simulink model "gm_DSBF"  (R2019b)
settings: Solver=FixedStepDiscrete  StartTime=0.0  StopTime=0.02  RelTol=1e-3
InitFcn:
  | sm_callback_init
StopFcn:
  | sm_callback_stop
undefined symbols (not defined in the file or in its folder): arraySize, arraySpacing, delayDataTypeFractionLength, delayDataTypeSign, delayDataTypeWordLength, mp, samplingRate, speedOfSound, upsampleFactor
libraries: hdlsllib x64, simulink x36, dspmlti4 x16, dsphdlfiltering x16
(part 4 of 5)

== system gm_DSBF/dataplane/Avalon Data Processing/delay signals_instance12/delay signal/read address generator ==
  note: To accommodate positive and negative delays, the read pointer needs to lag the write pointer by the maximum delay + 1. For the maximum positive delay, this puts the read pointer 1 behind the write pointer.
  note: this offset is the maximum possible delay from a microphone to the the center of the array
  note: wrap on overflow is the desired behavior
  write_addr : Inport  OutDataTypeStr=fixdt(0, 6, 0)  PortDimensions=1  SampleTime=2.08333333333333e-05
  delay : Inport  Port=2  OutDataTypeStr=fixdt(1, 6, 0)  PortDimensions=1  SampleTime=2.08333333333333e-05
  Increment Real World : simulink/Additional Math & Discrete/Additional Math: Increment - Decrement/Increment Real World
      settings: SourceProductName=Simulink  SourceProductBaseCode=SL
  Subtract : Subsystem
  phase center reference offset : Constant  Value=fix(mp.maxDelay/2)  OutDataTypeStr=fixdt(0,delayDataTypeWordLength - delayDataTypeFractionLength,0)  SampleTime=-1
  read_addr : Outport  VectorParamsAs1DForOutWhenUnconnected=off
  wires:
  delay/1 -> Subtract/1(In1)
  write_addr/1 -> Subtract/2(In2)
  Increment Real World/1 -> Subtract/3(In3)
  Subtract/1(Out1) -> read_addr/1
  phase center reference offset/1 -> Increment Real World/1

== system gm_DSBF/dataplane/Avalon Data Processing/delay signals_instance12/delay signal/read address generator1 ==
  note: wrap on overflow is the desired behavior
  note: To accommodate positive and negative delays, the read pointer needs to lag the write pointer by the maximum delay + 1. For the maximum positive delay, this puts the read pointer 1 behind the write pointer.
  note: this offset is the maximum possible delay from a microphone to the the center of the array
  write_addr : Inport  OutDataTypeStr=fixdt(0, 6, 0)  PortDimensions=1  SampleTime=1.30208333333333e-06
  delay : Inport  Port=2  OutDataTypeStr=fixdt(1, 6, 0)  PortDimensions=1  SampleTime=1.30208333333333e-06
  Increment Real World : simulink/Additional Math & Discrete/Additional Math: Increment - Decrement/Increment Real World
      settings: SourceProductName=Simulink  SourceProductBaseCode=SL
  Subtract : Subsystem
  phase center reference offset : Constant  Value=fix(mp.upsampleFactor)  OutDataTypeStr=fixdt(0, delayDataTypeFractionLength, 0)  SampleTime=-1
  read_addr : Outport  VectorParamsAs1DForOutWhenUnconnected=off
  wires:
  delay/1 -> Subtract/1(In1)
  write_addr/1 -> Subtract/2(In2)
  Increment Real World/1 -> Subtract/3(In3)
  Subtract/1(Out1) -> read_addr/1
  phase center reference offset/1 -> Increment Real World/1

== system gm_DSBF/dataplane/Avalon Data Processing/delay signals_instance12/delay signal/split_into_int_and_frac_parts ==
  delay : Inport  OutDataTypeStr=fixdt(1, 12, 6)  PortDimensions=1  SampleTime=2.08333333333333e-05
  split_into_int_and_frac_parts : MATLAB Function  TreatAsAtomicUnit=on
  integer_delay : Outport  VectorParamsAs1DForOutWhenUnconnected=off
  fractional_delay : Outport  Port=2
  wires:
  delay/1 -> split_into_int_and_frac_parts/1(delay)
  split_into_int_and_frac_parts/2(fractional_delay) -> fractional_delay/1
  split_into_int_and_frac_parts/1(integer_delay) -> integer_delay/1

== system gm_DSBF/dataplane/Avalon Data Processing/delay signals_instance13/delay signal/read address generator ==
  note: To accommodate positive and negative delays, the read pointer needs to lag the write pointer by the maximum delay + 1. For the maximum positive delay, this puts the read pointer 1 behind the write pointer.
  note: this offset is the maximum possible delay from a microphone to the the center of the array
  note: wrap on overflow is the desired behavior
  write_addr : Inport  OutDataTypeStr=fixdt(0, 6, 0)  PortDimensions=1  SampleTime=2.08333333333333e-05
  delay : Inport  Port=2  OutDataTypeStr=fixdt(1, 6, 0)  PortDimensions=1  SampleTime=2.08333333333333e-05
  Increment Real World : simulink/Additional Math & Discrete/Additional Math: Increment - Decrement/Increment Real World
      settings: SourceProductName=Simulink  SourceProductBaseCode=SL
  Subtract : Subsystem
  phase center reference offset : Constant  Value=fix(mp.maxDelay/2)  OutDataTypeStr=fixdt(0,delayDataTypeWordLength - delayDataTypeFractionLength,0)  SampleTime=-1
  read_addr : Outport  VectorParamsAs1DForOutWhenUnconnected=off
  wires:
  delay/1 -> Subtract/1(In1)
  write_addr/1 -> Subtract/2(In2)
  Increment Real World/1 -> Subtract/3(In3)
  Subtract/1(Out1) -> read_addr/1
  phase center reference offset/1 -> Increment Real World/1

== system gm_DSBF/dataplane/Avalon Data Processing/delay signals_instance13/delay signal/read address generator1 ==
  note: wrap on overflow is the desired behavior
  note: To accommodate positive and negative delays, the read pointer needs to lag the write pointer by the maximum delay + 1. For the maximum positive delay, this puts the read pointer 1 behind the write pointer.
  note: this offset is the maximum possible delay from a microphone to the the center of the array
  write_addr : Inport  OutDataTypeStr=fixdt(0, 6, 0)  PortDimensions=1  SampleTime=1.30208333333333e-06
  delay : Inport  Port=2  OutDataTypeStr=fixdt(1, 6, 0)  PortDimensions=1  SampleTime=1.30208333333333e-06
  Increment Real World : simulink/Additional Math & Discrete/Additional Math: Increment - Decrement/Increment Real World
      settings: SourceProductName=Simulink  SourceProductBaseCode=SL
  Subtract : Subsystem
  phase center reference offset : Constant  Value=fix(mp.upsampleFactor)  OutDataTypeStr=fixdt(0, delayDataTypeFractionLength, 0)  SampleTime=-1
  read_addr : Outport  VectorParamsAs1DForOutWhenUnconnected=off
  wires:
  delay/1 -> Subtract/1(In1)
  write_addr/1 -> Subtract/2(In2)
  Increment Real World/1 -> Subtract/3(In3)
  Subtract/1(Out1) -> read_addr/1
  phase center reference offset/1 -> Increment Real World/1

== system gm_DSBF/dataplane/Avalon Data Processing/delay signals_instance13/delay signal/split_into_int_and_frac_parts ==
  delay : Inport  OutDataTypeStr=fixdt(1, 12, 6)  PortDimensions=1  SampleTime=2.08333333333333e-05
  split_into_int_and_frac_parts : MATLAB Function  TreatAsAtomicUnit=on
  integer_delay : Outport  VectorParamsAs1DForOutWhenUnconnected=off
  fractional_delay : Outport  Port=2
  wires:
  delay/1 -> split_into_int_and_frac_parts/1(delay)
  split_into_int_and_frac_parts/2(fractional_delay) -> fractional_delay/1
  split_into_int_and_frac_parts/1(integer_delay) -> integer_delay/1

== system gm_DSBF/dataplane/Avalon Data Processing/delay signals_instance14/delay signal/read address generator ==
  note: To accommodate positive and negative delays, the read pointer needs to lag the write pointer by the maximum delay + 1. For the maximum positive delay, this puts the read pointer 1 behind the write pointer.
  note: this offset is the maximum possible delay from a microphone to the the center of the array
  note: wrap on overflow is the desired behavior
  write_addr : Inport  OutDataTypeStr=fixdt(0, 6, 0)  PortDimensions=1  SampleTime=2.08333333333333e-05
  delay : Inport  Port=2  OutDataTypeStr=fixdt(1, 6, 0)  PortDimensions=1  SampleTime=2.08333333333333e-05
  Increment Real World : simulink/Additional Math & Discrete/Additional Math: Increment - Decrement/Increment Real World
      settings: SourceProductName=Simulink  SourceProductBaseCode=SL
  Subtract : Subsystem
  phase center reference offset : Constant  Value=fix(mp.maxDelay/2)  OutDataTypeStr=fixdt(0,delayDataTypeWordLength - delayDataTypeFractionLength,0)  SampleTime=-1
  read_addr : Outport  VectorParamsAs1DForOutWhenUnconnected=off
  wires:
  delay/1 -> Subtract/1(In1)
  write_addr/1 -> Subtract/2(In2)
  Increment Real World/1 -> Subtract/3(In3)
  Subtract/1(Out1) -> read_addr/1
  phase center reference offset/1 -> Increment Real World/1

== system gm_DSBF/dataplane/Avalon Data Processing/delay signals_instance14/delay signal/read address generator1 ==
  note: wrap on overflow is the desired behavior
  note: To accommodate positive and negative delays, the read pointer needs to lag the write pointer by the maximum delay + 1. For the maximum positive delay, this puts the read pointer 1 behind the write pointer.
  note: this offset is the maximum possible delay from a microphone to the the center of the array
  write_addr : Inport  OutDataTypeStr=fixdt(0, 6, 0)  PortDimensions=1  SampleTime=1.30208333333333e-06
  delay : Inport  Port=2  OutDataTypeStr=fixdt(1, 6, 0)  PortDimensions=1  SampleTime=1.30208333333333e-06
  Increment Real World : simulink/Additional Math & Discrete/Additional Math: Increment - Decrement/Increment Real World
      settings: SourceProductName=Simulink  SourceProductBaseCode=SL
  Subtract : Subsystem
  phase center reference offset : Constant  Value=fix(mp.upsampleFactor)  OutDataTypeStr=fixdt(0, delayDataTypeFractionLength, 0)  SampleTime=-1
  read_addr : Outport  VectorParamsAs1DForOutWhenUnconnected=off
  wires:
  delay/1 -> Subtract/1(In1)
  write_addr/1 -> Subtract/2(In2)
  Increment Real World/1 -> Subtract/3(In3)
  Subtract/1(Out1) -> read_addr/1
  phase center reference offset/1 -> Increment Real World/1

== system gm_DSBF/dataplane/Avalon Data Processing/delay signals_instance14/delay signal/split_into_int_and_frac_parts ==
  delay : Inport  OutDataTypeStr=fixdt(1, 12, 6)  PortDimensions=1  SampleTime=2.08333333333333e-05
  split_into_int_and_frac_parts : MATLAB Function  TreatAsAtomicUnit=on
  integer_delay : Outport  VectorParamsAs1DForOutWhenUnconnected=off
  fractional_delay : Outport  Port=2
  wires:
  delay/1 -> split_into_int_and_frac_parts/1(delay)
  split_into_int_and_frac_parts/2(fractional_delay) -> fractional_delay/1
  split_into_int_and_frac_parts/1(integer_delay) -> integer_delay/1

== system gm_DSBF/dataplane/Avalon Data Processing/delay signals_instance15/delay signal/read address generator ==
  note: To accommodate positive and negative delays, the read pointer needs to lag the write pointer by the maximum delay + 1. For the maximum positive delay, this puts the read pointer 1 behind the write pointer.
  note: this offset is the maximum possible delay from a microphone to the the center of the array
  note: wrap on overflow is the desired behavior
  write_addr : Inport  OutDataTypeStr=fixdt(0, 6, 0)  PortDimensions=1  SampleTime=2.08333333333333e-05
  delay : Inport  Port=2  OutDataTypeStr=fixdt(1, 6, 0)  PortDimensions=1  SampleTime=2.08333333333333e-05
  Increment Real World : simulink/Additional Math & Discrete/Additional Math: Increment - Decrement/Increment Real World
      settings: SourceProductName=Simulink  SourceProductBaseCode=SL
  Subtract : Subsystem
  phase center reference offset : Constant  Value=fix(mp.maxDelay/2)  OutDataTypeStr=fixdt(0,delayDataTypeWordLength - delayDataTypeFractionLength,0)  SampleTime=-1
  read_addr : Outport  VectorParamsAs1DForOutWhenUnconnected=off
  wires:
  delay/1 -> Subtract/1(In1)
  write_addr/1 -> Subtract/2(In2)
  Increment Real World/1 -> Subtract/3(In3)
  Subtract/1(Out1) -> read_addr/1
  phase center reference offset/1 -> Increment Real World/1

== system gm_DSBF/dataplane/Avalon Data Processing/delay signals_instance15/delay signal/read address generator1 ==
  note: wrap on overflow is the desired behavior
  note: To accommodate positive and negative delays, the read pointer needs to lag the write pointer by the maximum delay + 1. For the maximum positive delay, this puts the read pointer 1 behind the write pointer.
  note: this offset is the maximum possible delay from a microphone to the the center of the array
  write_addr : Inport  OutDataTypeStr=fixdt(0, 6, 0)  PortDimensions=1  SampleTime=1.30208333333333e-06
  delay : Inport  Port=2  OutDataTypeStr=fixdt(1, 6, 0)  PortDimensions=1  SampleTime=1.30208333333333e-06
  Increment Real World : simulink/Additional Math & Discrete/Additional Math: Increment - Decrement/Increment Real World
      settings: SourceProductName=Simulink  SourceProductBaseCode=SL
  Subtract : Subsystem
  phase center reference offset : Constant  Value=fix(mp.upsampleFactor)  OutDataTypeStr=fixdt(0, delayDataTypeFractionLength, 0)  SampleTime=-1
  read_addr : Outport  VectorParamsAs1DForOutWhenUnconnected=off
  wires:
  delay/1 -> Subtract/1(In1)
  write_addr/1 -> Subtract/2(In2)
  Increment Real World/1 -> Subtract/3(In3)
  Subtract/1(Out1) -> read_addr/1
  phase center reference offset/1 -> Increment Real World/1

== system gm_DSBF/dataplane/Avalon Data Processing/delay signals_instance15/delay signal/split_into_int_and_frac_parts ==
  delay : Inport  OutDataTypeStr=fixdt(1, 12, 6)  PortDimensions=1  SampleTime=2.08333333333333e-05
  split_into_int_and_frac_parts : MATLAB Function  TreatAsAtomicUnit=on
  integer_delay : Outport  VectorParamsAs1DForOutWhenUnconnected=off
  fractional_delay : Outport  Port=2
  wires:
  delay/1 -> split_into_int_and_frac_parts/1(delay)
  split_into_int_and_frac_parts/2(fractional_delay) -> fractional_delay/1
  split_into_int_and_frac_parts/1(integer_delay) -> integer_delay/1

== system gm_DSBF/dataplane/Avalon Data Processing/delay signals_instance16/delay signal/read address generator ==
  note: To accommodate positive and negative delays, the read pointer needs to lag the write pointer by the maximum delay + 1. For the maximum positive delay, this puts the read pointer 1 behind the write pointer.
  note: this offset is the maximum possible delay from a microphone to the the center of the array
  note: wrap on overflow is the desired behavior
  write_addr : Inport  OutDataTypeStr=fixdt(0, 6, 0)  PortDimensions=1  SampleTime=2.08333333333333e-05
  delay : Inport  Port=2  OutDataTypeStr=fixdt(1, 6, 0)  PortDimensions=1  SampleTime=2.08333333333333e-05
  Increment Real World : simulink/Additional Math & Discrete/Additional Math: Increment - Decrement/Increment Real World
      settings: SourceProductName=Simulink  SourceProductBaseCode=SL
  Subtract : Subsystem
  phase center reference offset : Constant  Value=fix(mp.maxDelay/2)  OutDataTypeStr=fixdt(0,delayDataTypeWordLength - delayDataTypeFractionLength,0)  SampleTime=-1
  read_addr : Outport  VectorParamsAs1DForOutWhenUnconnected=off
  wires:
  delay/1 -> Subtract/1(In1)
  write_addr/1 -> Subtract/2(In2)
  Increment Real World/1 -> Subtract/3(In3)
  Subtract/1(Out1) -> read_addr/1
  phase center reference offset/1 -> Increment Real World/1

== system gm_DSBF/dataplane/Avalon Data Processing/delay signals_instance16/delay signal/read address generator1 ==
  note: wrap on overflow is the desired behavior
  note: To accommodate positive and negative delays, the read pointer needs to lag the write pointer by the maximum delay + 1. For the maximum positive delay, this puts the read pointer 1 behind the write pointer.
  note: this offset is the maximum possible delay from a microphone to the the center of the array
  write_addr : Inport  OutDataTypeStr=fixdt(0, 6, 0)  PortDimensions=1  SampleTime=1.30208333333333e-06
  delay : Inport  Port=2  OutDataTypeStr=fixdt(1, 6, 0)  PortDimensions=1  SampleTime=1.30208333333333e-06
  Increment Real World : simulink/Additional Math & Discrete/Additional Math: Increment - Decrement/Increment Real World
      settings: SourceProductName=Simulink  SourceProductBaseCode=SL
  Subtract : Subsystem
  phase center reference offset : Constant  Value=fix(mp.upsampleFactor)  OutDataTypeStr=fixdt(0, delayDataTypeFractionLength, 0)  SampleTime=-1
  read_addr : Outport  VectorParamsAs1DForOutWhenUnconnected=off
  wires:
  delay/1 -> Subtract/1(In1)
  write_addr/1 -> Subtract/2(In2)
  Increment Real World/1 -> Subtract/3(In3)
  Subtract/1(Out1) -> read_addr/1
  phase center reference offset/1 -> Increment Real World/1

== system gm_DSBF/dataplane/Avalon Data Processing/delay signals_instance16/delay signal/split_into_int_and_frac_parts ==
  delay : Inport  OutDataTypeStr=fixdt(1, 12, 6)  PortDimensions=1  SampleTime=2.08333333333333e-05
  split_into_int_and_frac_parts : MATLAB Function  TreatAsAtomicUnit=on
  integer_delay : Outport  VectorParamsAs1DForOutWhenUnconnected=off
  fractional_delay : Outport  Port=2
  wires:
  delay/1 -> split_into_int_and_frac_parts/1(delay)
  split_into_int_and_frac_parts/2(fractional_delay) -> fractional_delay/1
  split_into_int_and_frac_parts/1(integer_delay) -> integer_delay/1

== system gm_DSBF/dataplane/Avalon Data Processing/delay signals_instance2/delay signal/read address generator ==
  note: To accommodate positive and negative delays, the read pointer needs to lag the write pointer by the maximum delay + 1. For the maximum positive delay, this puts the read pointer 1 behind the write pointer.
  note: this offset is the maximum possible delay from a microphone to the the center of the array
  note: wrap on overflow is the desired behavior
  write_addr : Inport  OutDataTypeStr=fixdt(0, 6, 0)  PortDimensions=1  SampleTime=2.08333333333333e-05
  delay : Inport  Port=2  OutDataTypeStr=fixdt(1, 6, 0)  PortDimensions=1  SampleTime=2.08333333333333e-05
  Increment Real World : simulink/Additional Math & Discrete/Additional Math: Increment - Decrement/Increment Real World
      settings: SourceProductName=Simulink  SourceProductBaseCode=SL
  Subtract : Subsystem
  phase center reference offset : Constant  Value=fix(mp.maxDelay/2)  OutDataTypeStr=fixdt(0,delayDataTypeWordLength - delayDataTypeFractionLength,0)  SampleTime=-1
  read_addr : Outport  VectorParamsAs1DForOutWhenUnconnected=off
  wires:
  delay/1 -> Subtract/1(In1)
  write_addr/1 -> Subtract/2(In2)
  Increment Real World/1 -> Subtract/3(In3)
  Subtract/1(Out1) -> read_addr/1
  phase center reference offset/1 -> Increment Real World/1

== system gm_DSBF/dataplane/Avalon Data Processing/delay signals_instance2/delay signal/read address generator1 ==
  note: wrap on overflow is the desired behavior
  note: To accommodate positive and negative delays, the read pointer needs to lag the write pointer by the maximum delay + 1. For the maximum positive delay, this puts the read pointer 1 behind the write pointer.
  note: this offset is the maximum possible delay from a microphone to the the center of the array
  write_addr : Inport  OutDataTypeStr=fixdt(0, 6, 0)  PortDimensions=1  SampleTime=1.30208333333333e-06
  delay : Inport  Port=2  OutDataTypeStr=fixdt(1, 6, 0)  PortDimensions=1  SampleTime=1.30208333333333e-06
  Increment Real World : simulink/Additional Math & Discrete/Additional Math: Increment - Decrement/Increment Real World
      settings: SourceProductName=Simulink  SourceProductBaseCode=SL
  Subtract : Subsystem
  phase center reference offset : Constant  Value=fix(mp.upsampleFactor)  OutDataTypeStr=fixdt(0, delayDataTypeFractionLength, 0)  SampleTime=-1
  read_addr : Outport  VectorParamsAs1DForOutWhenUnconnected=off
  wires:
  delay/1 -> Subtract/1(In1)
  write_addr/1 -> Subtract/2(In2)
  Increment Real World/1 -> Subtract/3(In3)
  Subtract/1(Out1) -> read_addr/1
  phase center reference offset/1 -> Increment Real World/1

== system gm_DSBF/dataplane/Avalon Data Processing/delay signals_instance2/delay signal/split_into_int_and_frac_parts ==
  delay : Inport  OutDataTypeStr=fixdt(1, 12, 6)  PortDimensions=1  SampleTime=2.08333333333333e-05
  split_into_int_and_frac_parts : MATLAB Function  TreatAsAtomicUnit=on
  integer_delay : Outport  VectorParamsAs1DForOutWhenUnconnected=off
  fractional_delay : Outport  Port=2
  wires:
  delay/1 -> split_into_int_and_frac_parts/1(delay)
  split_into_int_and_frac_parts/2(fractional_delay) -> fractional_delay/1
  split_into_int_and_frac_parts/1(integer_delay) -> integer_delay/1

== system gm_DSBF/dataplane/Avalon Data Processing/delay signals_instance3/delay signal/read address generator ==
  note: To accommodate positive and negative delays, the read pointer needs to lag the write pointer by the maximum delay + 1. For the maximum positive delay, this puts the read pointer 1 behind the write pointer.
  note: this offset is the maximum possible delay from a microphone to the the center of the array
  note: wrap on overflow is the desired behavior
  write_addr : Inport  OutDataTypeStr=fixdt(0, 6, 0)  PortDimensions=1  SampleTime=2.08333333333333e-05
  delay : Inport  Port=2  OutDataTypeStr=fixdt(1, 6, 0)  PortDimensions=1  SampleTime=2.08333333333333e-05
  Increment Real World : simulink/Additional Math & Discrete/Additional Math: Increment - Decrement/Increment Real World
      settings: SourceProductName=Simulink  SourceProductBaseCode=SL
  Subtract : Subsystem
  phase center reference offset : Constant  Value=fix(mp.maxDelay/2)  OutDataTypeStr=fixdt(0,delayDataTypeWordLength - delayDataTypeFractionLength,0)  SampleTime=-1
  read_addr : Outport  VectorParamsAs1DForOutWhenUnconnected=off
  wires:
  delay/1 -> Subtract/1(In1)
  write_addr/1 -> Subtract/2(In2)
  Increment Real World/1 -> Subtract/3(In3)
  Subtract/1(Out1) -> read_addr/1
  phase center reference offset/1 -> Increment Real World/1

== system gm_DSBF/dataplane/Avalon Data Processing/delay signals_instance3/delay signal/read address generator1 ==
  note: wrap on overflow is the desired behavior
  note: To accommodate positive and negative delays, the read pointer needs to lag the write pointer by the maximum delay + 1. For the maximum positive delay, this puts the read pointer 1 behind the write pointer.
  note: this offset is the maximum possible delay from a microphone to the the center of the array
  write_addr : Inport  OutDataTypeStr=fixdt(0, 6, 0)  PortDimensions=1  SampleTime=1.30208333333333e-06
  delay : Inport  Port=2  OutDataTypeStr=fixdt(1, 6, 0)  PortDimensions=1  SampleTime=1.30208333333333e-06
  Increment Real World : simulink/Additional Math & Discrete/Additional Math: Increment - Decrement/Increment Real World
      settings: SourceProductName=Simulink  SourceProductBaseCode=SL
  Subtract : Subsystem
  phase center reference offset : Constant  Value=fix(mp.upsampleFactor)  OutDataTypeStr=fixdt(0, delayDataTypeFractionLength, 0)  SampleTime=-1
  read_addr : Outport  VectorParamsAs1DForOutWhenUnconnected=off
  wires:
  delay/1 -> Subtract/1(In1)
  write_addr/1 -> Subtract/2(In2)
  Increment Real World/1 -> Subtract/3(In3)
  Subtract/1(Out1) -> read_addr/1
  phase center reference offset/1 -> Increment Real World/1

== system gm_DSBF/dataplane/Avalon Data Processing/delay signals_instance3/delay signal/split_into_int_and_frac_parts ==
  delay : Inport  OutDataTypeStr=fixdt(1, 12, 6)  PortDimensions=1  SampleTime=2.08333333333333e-05
  split_into_int_and_frac_parts : MATLAB Function  TreatAsAtomicUnit=on
  integer_delay : Outport  VectorParamsAs1DForOutWhenUnconnected=off
  fractional_delay : Outport  Port=2
  wires:
  delay/1 -> split_into_int_and_frac_parts/1(delay)
  split_into_int_and_frac_parts/2(fractional_delay) -> fractional_delay/1
  split_into_int_and_frac_parts/1(integer_delay) -> integer_delay/1

== system gm_DSBF/dataplane/Avalon Data Processing/delay signals_instance4/delay signal/read address generator ==
  note: To accommodate positive and negative delays, the read pointer needs to lag the write pointer by the maximum delay + 1. For the maximum positive delay, this puts the read pointer 1 behind the write pointer.
  note: this offset is the maximum possible delay from a microphone to the the center of the array
  note: wrap on overflow is the desired behavior
  write_addr : Inport  OutDataTypeStr=fixdt(0, 6, 0)  PortDimensions=1  SampleTime=2.08333333333333e-05
  delay : Inport  Port=2  OutDataTypeStr=fixdt(1, 6, 0)  PortDimensions=1  SampleTime=2.08333333333333e-05
  Increment Real World : simulink/Additional Math & Discrete/Additional Math: Increment - Decrement/Increment Real World
      settings: SourceProductName=Simulink  SourceProductBaseCode=SL
  Subtract : Subsystem
  phase center reference offset : Constant  Value=fix(mp.maxDelay/2)  OutDataTypeStr=fixdt(0,delayDataTypeWordLength - delayDataTypeFractionLength,0)  SampleTime=-1
  read_addr : Outport  VectorParamsAs1DForOutWhenUnconnected=off
  wires:
  delay/1 -> Subtract/1(In1)
  write_addr/1 -> Subtract/2(In2)
  Increment Real World/1 -> Subtract/3(In3)
  Subtract/1(Out1) -> read_addr/1
  phase center reference offset/1 -> Increment Real World/1

== system gm_DSBF/dataplane/Avalon Data Processing/delay signals_instance4/delay signal/read address generator1 ==
  note: wrap on overflow is the desired behavior
  note: To accommodate positive and negative delays, the read pointer needs to lag the write pointer by the maximum delay + 1. For the maximum positive delay, this puts the read pointer 1 behind the write pointer.
  note: this offset is the maximum possible delay from a microphone to the the center of the array
  write_addr : Inport  OutDataTypeStr=fixdt(0, 6, 0)  PortDimensions=1  SampleTime=1.30208333333333e-06
  delay : Inport  Port=2  OutDataTypeStr=fixdt(1, 6, 0)  PortDimensions=1  SampleTime=1.30208333333333e-06
  Increment Real World : simulink/Additional Math & Discrete/Additional Math: Increment - Decrement/Increment Real World
      settings: SourceProductName=Simulink  SourceProductBaseCode=SL
  Subtract : Subsystem
  phase center reference offset : Constant  Value=fix(mp.upsampleFactor)  OutDataTypeStr=fixdt(0, delayDataTypeFractionLength, 0)  SampleTime=-1
  read_addr : Outport  VectorParamsAs1DForOutWhenUnconnected=off
  wires:
  delay/1 -> Subtract/1(In1)
  write_addr/1 -> Subtract/2(In2)
  Increment Real World/1 -> Subtract/3(In3)
  Subtract/1(Out1) -> read_addr/1
  phase center reference offset/1 -> Increment Real World/1

== system gm_DSBF/dataplane/Avalon Data Processing/delay signals_instance4/delay signal/split_into_int_and_frac_parts ==
  delay : Inport  OutDataTypeStr=fixdt(1, 12, 6)  PortDimensions=1  SampleTime=2.08333333333333e-05
  split_into_int_and_frac_parts : MATLAB Function  TreatAsAtomicUnit=on
  integer_delay : Outport  VectorParamsAs1DForOutWhenUnconnected=off
  fractional_delay : Outport  Port=2
  wires:
  delay/1 -> split_into_int_and_frac_parts/1(delay)
  split_into_int_and_frac_parts/2(fractional_delay) -> fractional_delay/1
  split_into_int_and_frac_parts/1(integer_delay) -> integer_delay/1

== system gm_DSBF/dataplane/Avalon Data Processing/delay signals_instance5/delay signal/read address generator ==
  note: To accommodate positive and negative delays, the read pointer needs to lag the write pointer by the maximum delay + 1. For the maximum positive delay, this puts the read pointer 1 behind the write pointer.
  note: this offset is the maximum possible delay from a microphone to the the center of the array
  note: wrap on overflow is the desired behavior
  write_addr : Inport  OutDataTypeStr=fixdt(0, 6, 0)  PortDimensions=1  SampleTime=2.08333333333333e-05
  delay : Inport  Port=2  OutDataTypeStr=fixdt(1, 6, 0)  PortDimensions=1  SampleTime=2.08333333333333e-05
  Increment Real World : simulink/Additional Math & Discrete/Additional Math: Increment - Decrement/Increment Real World
      settings: SourceProductName=Simulink  SourceProductBaseCode=SL
  Subtract : Subsystem
  phase center reference offset : Constant  Value=fix(mp.maxDelay/2)  OutDataTypeStr=fixdt(0,delayDataTypeWordLength - delayDataTypeFractionLength,0)  SampleTime=-1
  read_addr : Outport  VectorParamsAs1DForOutWhenUnconnected=off
  wires:
  delay/1 -> Subtract/1(In1)
  write_addr/1 -> Subtract/2(In2)
  Increment Real World/1 -> Subtract/3(In3)
  Subtract/1(Out1) -> read_addr/1
  phase center reference offset/1 -> Increment Real World/1

== system gm_DSBF/dataplane/Avalon Data Processing/delay signals_instance5/delay signal/read address generator1 ==
  note: wrap on overflow is the desired behavior
  note: To accommodate positive and negative delays, the read pointer needs to lag the write pointer by the maximum delay + 1. For the maximum positive delay, this puts the read pointer 1 behind the write pointer.
  note: this offset is the maximum possible delay from a microphone to the the center of the array
  write_addr : Inport  OutDataTypeStr=fixdt(0, 6, 0)  PortDimensions=1  SampleTime=1.30208333333333e-06
  delay : Inport  Port=2  OutDataTypeStr=fixdt(1, 6, 0)  PortDimensions=1  SampleTime=1.30208333333333e-06
  Increment Real World : simulink/Additional Math & Discrete/Additional Math: Increment - Decrement/Increment Real World
      settings: SourceProductName=Simulink  SourceProductBaseCode=SL
  Subtract : Subsystem
  phase center reference offset : Constant  Value=fix(mp.upsampleFactor)  OutDataTypeStr=fixdt(0, delayDataTypeFractionLength, 0)  SampleTime=-1
  read_addr : Outport  VectorParamsAs1DForOutWhenUnconnected=off
  wires:
  delay/1 -> Subtract/1(In1)
  write_addr/1 -> Subtract/2(In2)
  Increment Real World/1 -> Subtract/3(In3)
  Subtract/1(Out1) -> read_addr/1
  phase center reference offset/1 -> Increment Real World/1

== system gm_DSBF/dataplane/Avalon Data Processing/delay signals_instance5/delay signal/split_into_int_and_frac_parts ==
  delay : Inport  OutDataTypeStr=fixdt(1, 12, 6)  PortDimensions=1  SampleTime=2.08333333333333e-05
  split_into_int_and_frac_parts : MATLAB Function  TreatAsAtomicUnit=on
  integer_delay : Outport  VectorParamsAs1DForOutWhenUnconnected=off
  fractional_delay : Outport  Port=2
  wires:
  delay/1 -> split_into_int_and_frac_parts/1(delay)
  split_into_int_and_frac_parts/2(fractional_delay) -> fractional_delay/1
  split_into_int_and_frac_parts/1(integer_delay) -> integer_delay/1

== system gm_DSBF/dataplane/Avalon Data Processing/delay signals_instance6/delay signal/read address generator ==
  note: To accommodate positive and negative delays, the read pointer needs to lag the write pointer by the maximum delay + 1. For the maximum positive delay, this puts the read pointer 1 behind the write pointer.
  note: this offset is the maximum possible delay from a microphone to the the center of the array
  note: wrap on overflow is the desired behavior
  write_addr : Inport  OutDataTypeStr=fixdt(0, 6, 0)  PortDimensions=1  SampleTime=2.08333333333333e-05
  delay : Inport  Port=2  OutDataTypeStr=fixdt(1, 6, 0)  PortDimensions=1  SampleTime=2.08333333333333e-05
  Increment Real World : simulink/Additional Math & Discrete/Additional Math: Increment - Decrement/Increment Real World
      settings: SourceProductName=Simulink  SourceProductBaseCode=SL
  Subtract : Subsystem
  phase center reference offset : Constant  Value=fix(mp.maxDelay/2)  OutDataTypeStr=fixdt(0,delayDataTypeWordLength - delayDataTypeFractionLength,0)  SampleTime=-1
  read_addr : Outport  VectorParamsAs1DForOutWhenUnconnected=off
  wires:
  delay/1 -> Subtract/1(In1)
  write_addr/1 -> Subtract/2(In2)
  Increment Real World/1 -> Subtract/3(In3)
  Subtract/1(Out1) -> read_addr/1
  phase center reference offset/1 -> Increment Real World/1

== system gm_DSBF/dataplane/Avalon Data Processing/delay signals_instance6/delay signal/read address generator1 ==
  note: wrap on overflow is the desired behavior
  note: To accommodate positive and negative delays, the read pointer needs to lag the write pointer by the maximum delay + 1. For the maximum positive delay, this puts the read pointer 1 behind the write pointer.
  note: this offset is the maximum possible delay from a microphone to the the center of the array
  write_addr : Inport  OutDataTypeStr=fixdt(0, 6, 0)  PortDimensions=1  SampleTime=1.30208333333333e-06
  delay : Inport  Port=2  OutDataTypeStr=fixdt(1, 6, 0)  PortDimensions=1  SampleTime=1.30208333333333e-06
  Increment Real World : simulink/Additional Math & Discrete/Additional Math: Increment - Decrement/Increment Real World
      settings: SourceProductName=Simulink  SourceProductBaseCode=SL
  Subtract : Subsystem
  phase center reference offset : Constant  Value=fix(mp.upsampleFactor)  OutDataTypeStr=fixdt(0, delayDataTypeFractionLength, 0)  SampleTime=-1
  read_addr : Outport  VectorParamsAs1DForOutWhenUnconnected=off
  wires:
  delay/1 -> Subtract/1(In1)
  write_addr/1 -> Subtract/2(In2)
  Increment Real World/1 -> Subtract/3(In3)
  Subtract/1(Out1) -> read_addr/1
  phase center reference offset/1 -> Increment Real World/1

== system gm_DSBF/dataplane/Avalon Data Processing/delay signals_instance6/delay signal/split_into_int_and_frac_parts ==
  delay : Inport  OutDataTypeStr=fixdt(1, 12, 6)  PortDimensions=1  SampleTime=2.08333333333333e-05
  split_into_int_and_frac_parts : MATLAB Function  TreatAsAtomicUnit=on
  integer_delay : Outport  VectorParamsAs1DForOutWhenUnconnected=off
  fractional_delay : Outport  Port=2
  wires:
  delay/1 -> split_into_int_and_frac_parts/1(delay)
  split_into_int_and_frac_parts/2(fractional_delay) -> fractional_delay/1
  split_into_int_and_frac_parts/1(integer_delay) -> integer_delay/1

== system gm_DSBF/dataplane/Avalon Data Processing/delay signals_instance7/delay signal/read address generator ==
  note: To accommodate positive and negative delays, the read pointer needs to lag the write pointer by the maximum delay + 1. For the maximum positive delay, this puts the read pointer 1 behind the write pointer.
  note: this offset is the maximum possible delay from a microphone to the the center of the array
  note: wrap on overflow is the desired behavior
  write_addr : Inport  OutDataTypeStr=fixdt(0, 6, 0)  PortDimensions=1  SampleTime=2.08333333333333e-05
  delay : Inport  Port=2  OutDataTypeStr=fixdt(1, 6, 0)  PortDimensions=1  SampleTime=2.08333333333333e-05
  Increment Real World : simulink/Additional Math & Discrete/Additional Math: Increment - Decrement/Increment Real World
      settings: SourceProductName=Simulink  SourceProductBaseCode=SL
  Subtract : Subsystem
  phase center reference offset : Constant  Value=fix(mp.maxDelay/2)  OutDataTypeStr=fixdt(0,delayDataTypeWordLength - delayDataTypeFractionLength,0)  SampleTime=-1
  read_addr : Outport  VectorParamsAs1DForOutWhenUnconnected=off
  wires:
  delay/1 -> Subtract/1(In1)
  write_addr/1 -> Subtract/2(In2)
  Increment Real World/1 -> Subtract/3(In3)
  Subtract/1(Out1) -> read_addr/1
  phase center reference offset/1 -> Increment Real World/1

== system gm_DSBF/dataplane/Avalon Data Processing/delay signals_instance7/delay signal/read address generator1 ==
  note: wrap on overflow is the desired behavior
  note: To accommodate positive and negative delays, the read pointer needs to lag the write pointer by the maximum delay + 1. For the maximum positive delay, this puts the read pointer 1 behind the write pointer.
  note: this offset is the maximum possible delay from a microphone to the the center of the array
  write_addr : Inport  OutDataTypeStr=fixdt(0, 6, 0)  PortDimensions=1  SampleTime=1.30208333333333e-06
  delay : Inport  Port=2  OutDataTypeStr=fixdt(1, 6, 0)  PortDimensions=1  SampleTime=1.30208333333333e-06
  Increment Real World : simulink/Additional Math & Discrete/Additional Math: Increment - Decrement/Increment Real World
      settings: SourceProductName=Simulink  SourceProductBaseCode=SL
  Subtract : Subsystem
  phase center reference offset : Constant  Value=fix(mp.upsampleFactor)  OutDataTypeStr=fixdt(0, delayDataTypeFractionLength, 0)  SampleTime=-1
  read_addr : Outport  VectorParamsAs1DForOutWhenUnconnected=off
  wires:
  delay/1 -> Subtract/1(In1)
  write_addr/1 -> Subtract/2(In2)
  Increment Real World/1 -> Subtract/3(In3)
  Subtract/1(Out1) -> read_addr/1
  phase center reference offset/1 -> Increment Real World/1

== system gm_DSBF/dataplane/Avalon Data Processing/delay signals_instance7/delay signal/split_into_int_and_frac_parts ==
  delay : Inport  OutDataTypeStr=fixdt(1, 12, 6)  PortDimensions=1  SampleTime=2.08333333333333e-05
  split_into_int_and_frac_parts : MATLAB Function  TreatAsAtomicUnit=on
  integer_delay : Outport  VectorParamsAs1DForOutWhenUnconnected=off
  fractional_delay : Outport  Port=2
  wires:
  delay/1 -> split_into_int_and_frac_parts/1(delay)
  split_into_int_and_frac_parts/2(fractional_delay) -> fractional_delay/1
  split_into_int_and_frac_parts/1(integer_delay) -> integer_delay/1

== system gm_DSBF/dataplane/Avalon Data Processing/delay signals_instance8/delay signal/read address generator ==
  note: To accommodate positive and negative delays, the read pointer needs to lag the write pointer by the maximum delay + 1. For the maximum positive delay, this puts the read pointer 1 behind the write pointer.
  note: this offset is the maximum possible delay from a microphone to the the center of the array
  note: wrap on overflow is the desired behavior
  write_addr : Inport  OutDataTypeStr=fixdt(0, 6, 0)  PortDimensions=1  SampleTime=2.08333333333333e-05
  delay : Inport  Port=2  OutDataTypeStr=fixdt(1, 6, 0)  PortDimensions=1  SampleTime=2.08333333333333e-05
  Increment Real World : simulink/Additional Math & Discrete/Additional Math: Increment - Decrement/Increment Real World
      settings: SourceProductName=Simulink  SourceProductBaseCode=SL
  Subtract : Subsystem
  phase center reference offset : Constant  Value=fix(mp.maxDelay/2)  OutDataTypeStr=fixdt(0,delayDataTypeWordLength - delayDataTypeFractionLength,0)  SampleTime=-1
  read_addr : Outport  VectorParamsAs1DForOutWhenUnconnected=off
  wires:
  delay/1 -> Subtract/1(In1)
  write_addr/1 -> Subtract/2(In2)
  Increment Real World/1 -> Subtract/3(In3)
  Subtract/1(Out1) -> read_addr/1
  phase center reference offset/1 -> Increment Real World/1

== system gm_DSBF/dataplane/Avalon Data Processing/delay signals_instance8/delay signal/read address generator1 ==
  note: wrap on overflow is the desired behavior
  note: To accommodate positive and negative delays, the read pointer needs to lag the write pointer by the maximum delay + 1. For the maximum positive delay, this puts the read pointer 1 behind the write pointer.
  note: this offset is the maximum possible delay from a microphone to the the center of the array
  write_addr : Inport  OutDataTypeStr=fixdt(0, 6, 0)  PortDimensions=1  SampleTime=1.30208333333333e-06
  delay : Inport  Port=2  OutDataTypeStr=fixdt(1, 6, 0)  PortDimensions=1  SampleTime=1.30208333333333e-06
  Increment Real World : simulink/Additional Math & Discrete/Additional Math: Increment - Decrement/Increment Real World
      settings: SourceProductName=Simulink  SourceProductBaseCode=SL
  Subtract : Subsystem
  phase center reference offset : Constant  Value=fix(mp.upsampleFactor)  OutDataTypeStr=fixdt(0, delayDataTypeFractionLength, 0)  SampleTime=-1
  read_addr : Outport  VectorParamsAs1DForOutWhenUnconnected=off
  wires:
  delay/1 -> Subtract/1(In1)
  write_addr/1 -> Subtract/2(In2)
  Increment Real World/1 -> Subtract/3(In3)
  Subtract/1(Out1) -> read_addr/1
  phase center reference offset/1 -> Increment Real World/1

== system gm_DSBF/dataplane/Avalon Data Processing/delay signals_instance8/delay signal/split_into_int_and_frac_parts ==
  delay : Inport  OutDataTypeStr=fixdt(1, 12, 6)  PortDimensions=1  SampleTime=2.08333333333333e-05
  split_into_int_and_frac_parts : MATLAB Function  TreatAsAtomicUnit=on
  integer_delay : Outport  VectorParamsAs1DForOutWhenUnconnected=off
  fractional_delay : Outport  Port=2
  wires:
  delay/1 -> split_into_int_and_frac_parts/1(delay)
  split_into_int_and_frac_parts/2(fractional_delay) -> fractional_delay/1
  split_into_int_and_frac_parts/1(integer_delay) -> integer_delay/1

== system gm_DSBF/dataplane/Avalon Data Processing/delay signals_instance9/delay signal/read address generator ==
  note: To accommodate positive and negative delays, the read pointer needs to lag the write pointer by the maximum delay + 1. For the maximum positive delay, this puts the read pointer 1 behind the write pointer.
  note: this offset is the maximum possible delay from a microphone to the the center of the array
  note: wrap on overflow is the desired behavior
  write_addr : Inport  OutDataTypeStr=fixdt(0, 6, 0)  PortDimensions=1  SampleTime=2.08333333333333e-05
  delay : Inport  Port=2  OutDataTypeStr=fixdt(1, 6, 0)  PortDimensions=1  SampleTime=2.08333333333333e-05
  Increment Real World : simulink/Additional Math & Discrete/Additional Math: Increment - Decrement/Increment Real World
      settings: SourceProductName=Simulink  SourceProductBaseCode=SL
  Subtract : Subsystem
  phase center reference offset : Constant  Value=fix(mp.maxDelay/2)  OutDataTypeStr=fixdt(0,delayDataTypeWordLength - delayDataTypeFractionLength,0)  SampleTime=-1
  read_addr : Outport  VectorParamsAs1DForOutWhenUnconnected=off
  wires:
  delay/1 -> Subtract/1(In1)
  write_addr/1 -> Subtract/2(In2)
  Increment Real World/1 -> Subtract/3(In3)
  Subtract/1(Out1) -> read_addr/1
  phase center reference offset/1 -> Increment Real World/1

== system gm_DSBF/dataplane/Avalon Data Processing/delay signals_instance9/delay signal/read address generator1 ==
  note: wrap on overflow is the desired behavior
  note: To accommodate positive and negative delays, the read pointer needs to lag the write pointer by the maximum delay + 1. For the maximum positive delay, this puts the read pointer 1 behind the write pointer.
  note: this offset is the maximum possible delay from a microphone to the the center of the array
  write_addr : Inport  OutDataTypeStr=fixdt(0, 6, 0)  PortDimensions=1  SampleTime=1.30208333333333e-06
  delay : Inport  Port=2  OutDataTypeStr=fixdt(1, 6, 0)  PortDimensions=1  SampleTime=1.30208333333333e-06
  Increment Real World : simulink/Additional Math & Discrete/Additional Math: Increment - Decrement/Increment Real World
      settings: SourceProductName=Simulink  SourceProductBaseCode=SL
  Subtract : Subsystem
  phase center reference offset : Constant  Value=fix(mp.upsampleFactor)  OutDataTypeStr=fixdt(0, delayDataTypeFractionLength, 0)  SampleTime=-1
  read_addr : Outport  VectorParamsAs1DForOutWhenUnconnected=off
  wires:
  delay/1 -> Subtract/1(In1)
  write_addr/1 -> Subtract/2(In2)
  Increment Real World/1 -> Subtract/3(In3)
  Subtract/1(Out1) -> read_addr/1
  phase center reference offset/1 -> Increment Real World/1

== system gm_DSBF/dataplane/Avalon Data Processing/delay signals_instance9/delay signal/split_into_int_and_frac_parts ==
  delay : Inport  OutDataTypeStr=fixdt(1, 12, 6)  PortDimensions=1  SampleTime=2.08333333333333e-05
  split_into_int_and_frac_parts : MATLAB Function  TreatAsAtomicUnit=on
  integer_delay : Outport  VectorParamsAs1DForOutWhenUnconnected=off
  fractional_delay : Outport  Port=2
  wires:
  delay/1 -> split_into_int_and_frac_parts/1(delay)
  split_into_int_and_frac_parts/2(fractional_delay) -> fractional_delay/1
  split_into_int_and_frac_parts/1(integer_delay) -> integer_delay/1

== system gm_DSBF/dataplane/Avalon Data Processing/delay signals_instance1/delay signal/read address generator/Subtract ==
  In1 : Inport  OutDataTypeStr=fixdt(1,6,0)
  In2 : Inport  Port=2  OutDataTypeStr=fixdt(0,6,0)
  In3 : Inport  Port=3  OutDataTypeStr=fixdt(0,6,0)
  Sum2 : Sum  AccumDataTypeStr=fixdt(1,8,0)  OutDataTypeStr=fixdt(1,8,0)
  Sum3 : Sum  Inputs=+-  AccumDataTypeStr=fixdt(1,8,0)  OutDataTypeStr=fixdt(0,6,0)
  Out1 : Outport
  wires:
  In1/1 -> Sum2/1
  In2/1 -> Sum2/2
  Sum2/1 -> Sum3/1
  In3/1 -> Sum3/2
  Sum3/1 -> Out1/1

== system gm_DSBF/dataplane/Avalon Data Processing/delay signals_instance1/delay signal/read address generator1/Subtract ==
  In1 : Inport  OutDataTypeStr=fixdt(1,6,0)
  In2 : Inport  Port=2  OutDataTypeStr=fixdt(0,6,0)
  In3 : Inport  Port=3  OutDataTypeStr=fixdt(0,6,0)
  Sum2 : Sum  AccumDataTypeStr=fixdt(1,8,0)  OutDataTypeStr=fixdt(1,8,0)
  Sum3 : Sum  Inputs=+-  AccumDataTypeStr=fixdt(1,8,0)  OutDataTypeStr=fixdt(0,6,0)
  Out1 : Outport
  wires:
  In1/1 -> Sum2/1
  In2/1 -> Sum2/2
  Sum2/1 -> Sum3/1
  In3/1 -> Sum3/2
  Sum3/1 -> Out1/1

== system gm_DSBF/dataplane/Avalon Data Processing/delay signals_instance10/delay signal/read address generator/Subtract ==
  In1 : Inport  OutDataTypeStr=fixdt(1,6,0)
  In2 : Inport  Port=2  OutDataTypeStr=fixdt(0,6,0)
  In3 : Inport  Port=3  OutDataTypeStr=fixdt(0,6,0)
  Sum2 : Sum  AccumDataTypeStr=fixdt(1,8,0)  OutDataTypeStr=fixdt(1,8,0)
  Sum3 : Sum  Inputs=+-  AccumDataTypeStr=fixdt(1,8,0)  OutDataTypeStr=fixdt(0,6,0)
  Out1 : Outport
  wires:
  Sum3/1 -> Out1/1
  In3/1 -> Sum3/2
  Sum2/1 -> Sum3/1
  In2/1 -> Sum2/2
  In1/1 -> Sum2/1

== system gm_DSBF/dataplane/Avalon Data Processing/delay signals_instance10/delay signal/read address generator1/Subtract ==
  In1 : Inport  OutDataTypeStr=fixdt(1,6,0)
  In2 : Inport  Port=2  OutDataTypeStr=fixdt(0,6,0)
  In3 : Inport  Port=3  OutDataTypeStr=fixdt(0,6,0)
  Sum2 : Sum  AccumDataTypeStr=fixdt(1,8,0)  OutDataTypeStr=fixdt(1,8,0)
  Sum3 : Sum  Inputs=+-  AccumDataTypeStr=fixdt(1,8,0)  OutDataTypeStr=fixdt(0,6,0)
  Out1 : Outport
  wires:
  Sum3/1 -> Out1/1
  In3/1 -> Sum3/2
  Sum2/1 -> Sum3/1
  In2/1 -> Sum2/2
  In1/1 -> Sum2/1

== system gm_DSBF/dataplane/Avalon Data Processing/delay signals_instance11/delay signal/read address generator/Subtract ==
  In1 : Inport  OutDataTypeStr=fixdt(1,6,0)
  In2 : Inport  Port=2  OutDataTypeStr=fixdt(0,6,0)
  In3 : Inport  Port=3  OutDataTypeStr=fixdt(0,6,0)
  Sum2 : Sum  AccumDataTypeStr=fixdt(1,8,0)  OutDataTypeStr=fixdt(1,8,0)
  Sum3 : Sum  Inputs=+-  AccumDataTypeStr=fixdt(1,8,0)  OutDataTypeStr=fixdt(0,6,0)
  Out1 : Outport
  wires:
  Sum3/1 -> Out1/1
  In3/1 -> Sum3/2
  Sum2/1 -> Sum3/1
  In2/1 -> Sum2/2
  In1/1 -> Sum2/1

== system gm_DSBF/dataplane/Avalon Data Processing/delay signals_instance11/delay signal/read address generator1/Subtract ==
  In1 : Inport  OutDataTypeStr=fixdt(1,6,0)
  In2 : Inport  Port=2  OutDataTypeStr=fixdt(0,6,0)
  In3 : Inport  Port=3  OutDataTypeStr=fixdt(0,6,0)
  Sum2 : Sum  AccumDataTypeStr=fixdt(1,8,0)  OutDataTypeStr=fixdt(1,8,0)
  Sum3 : Sum  Inputs=+-  AccumDataTypeStr=fixdt(1,8,0)  OutDataTypeStr=fixdt(0,6,0)
  Out1 : Outport
  wires:
  Sum3/1 -> Out1/1
  In3/1 -> Sum3/2
  Sum2/1 -> Sum3/1
  In2/1 -> Sum2/2
  In1/1 -> Sum2/1

== system gm_DSBF/dataplane/Avalon Data Processing/delay signals_instance12/delay signal/read address generator/Subtract ==
  In1 : Inport  OutDataTypeStr=fixdt(1,6,0)
  In2 : Inport  Port=2  OutDataTypeStr=fixdt(0,6,0)
  In3 : Inport  Port=3  OutDataTypeStr=fixdt(0,6,0)
  Sum2 : Sum  AccumDataTypeStr=fixdt(1,8,0)  OutDataTypeStr=fixdt(1,8,0)
  Sum3 : Sum  Inputs=+-  AccumDataTypeStr=fixdt(1,8,0)  OutDataTypeStr=fixdt(0,6,0)
  Out1 : Outport
  wires:
  Sum3/1 -> Out1/1
  In3/1 -> Sum3/2
  Sum2/1 -> Sum3/1
  In2/1 -> Sum2/2
  In1/1 -> Sum2/1

== system gm_DSBF/dataplane/Avalon Data Processing/delay signals_instance12/delay signal/read address generator1/Subtract ==
  In1 : Inport  OutDataTypeStr=fixdt(1,6,0)
  In2 : Inport  Port=2  OutDataTypeStr=fixdt(0,6,0)
  In3 : Inport  Port=3  OutDataTypeStr=fixdt(0,6,0)
  Sum2 : Sum  AccumDataTypeStr=fixdt(1,8,0)  OutDataTypeStr=fixdt(1,8,0)
  Sum3 : Sum  Inputs=+-  AccumDataTypeStr=fixdt(1,8,0)  OutDataTypeStr=fixdt(0,6,0)
  Out1 : Outport
  wires:
  Sum3/1 -> Out1/1
  In3/1 -> Sum3/2
  Sum2/1 -> Sum3/1
  In2/1 -> Sum2/2
  In1/1 -> Sum2/1

== system gm_DSBF/dataplane/Avalon Data Processing/delay signals_instance13/delay signal/read address generator/Subtract ==
  In1 : Inport  OutDataTypeStr=fixdt(1,6,0)
  In2 : Inport  Port=2  OutDataTypeStr=fixdt(0,6,0)
  In3 : Inport  Port=3  OutDataTypeStr=fixdt(0,6,0)
  Sum2 : Sum  AccumDataTypeStr=fixdt(1,8,0)  OutDataTypeStr=fixdt(1,8,0)
  Sum3 : Sum  Inputs=+-  AccumDataTypeStr=fixdt(1,8,0)  OutDataTypeStr=fixdt(0,6,0)
  Out1 : Outport
  wires:
  Sum3/1 -> Out1/1
  In3/1 -> Sum3/2
  Sum2/1 -> Sum3/1
  In2/1 -> Sum2/2
  In1/1 -> Sum2/1

== system gm_DSBF/dataplane/Avalon Data Processing/delay signals_instance13/delay signal/read address generator1/Subtract ==
  In1 : Inport  OutDataTypeStr=fixdt(1,6,0)
  In2 : Inport  Port=2  OutDataTypeStr=fixdt(0,6,0)
  In3 : Inport  Port=3  OutDataTypeStr=fixdt(0,6,0)
  Sum2 : Sum  AccumDataTypeStr=fixdt(1,8,0)  OutDataTypeStr=fixdt(1,8,0)
  Sum3 : Sum  Inputs=+-  AccumDataTypeStr=fixdt(1,8,0)  OutDataTypeStr=fixdt(0,6,0)
  Out1 : Outport
  wires:
  Sum3/1 -> Out1/1
  In3/1 -> Sum3/2
  Sum2/1 -> Sum3/1
  In2/1 -> Sum2/2
  In1/1 -> Sum2/1

== system gm_DSBF/dataplane/Avalon Data Processing/delay signals_instance14/delay signal/read address generator/Subtract ==
  In1 : Inport  OutDataTypeStr=fixdt(1,6,0)
  In2 : Inport  Port=2  OutDataTypeStr=fixdt(0,6,0)
  In3 : Inport  Port=3  OutDataTypeStr=fixdt(0,6,0)
  Sum2 : Sum  AccumDataTypeStr=fixdt(1,8,0)  OutDataTypeStr=fixdt(1,8,0)
  Sum3 : Sum  Inputs=+-  AccumDataTypeStr=fixdt(1,8,0)  OutDataTypeStr=fixdt(0,6,0)
  Out1 : Outport
  wires:
  Sum3/1 -> Out1/1
  In3/1 -> Sum3/2
  Sum2/1 -> Sum3/1
  In2/1 -> Sum2/2
  In1/1 -> Sum2/1

== system gm_DSBF/dataplane/Avalon Data Processing/delay signals_instance14/delay signal/read address generator1/Subtract ==
  In1 : Inport  OutDataTypeStr=fixdt(1,6,0)
  In2 : Inport  Port=2  OutDataTypeStr=fixdt(0,6,0)
  In3 : Inport  Port=3  OutDataTypeStr=fixdt(0,6,0)
  Sum2 : Sum  AccumDataTypeStr=fixdt(1,8,0)  OutDataTypeStr=fixdt(1,8,0)
  Sum3 : Sum  Inputs=+-  AccumDataTypeStr=fixdt(1,8,0)  OutDataTypeStr=fixdt(0,6,0)
  Out1 : Outport
  wires:
  Sum3/1 -> Out1/1
  In3/1 -> Sum3/2
  Sum2/1 -> Sum3/1
  In2/1 -> Sum2/2
  In1/1 -> Sum2/1
